simulink model "TST_AdvancedStateflowLoops4"  (Simulink 7.8)
settings: Solver=FixedStepDiscrete  StartTime=0.0  StopTime=10.0  FixedStep=0.02  RelTol=1e-3
settings Model: Creator=kharthforeign  LastModifiedBy=kharthforeign  BufferReuse=off
settings DataIOCC: SaveOutput=off  SignalLogging=off  SaveTime=off
settings OptimizationCC: BlockReduction=off  ConditionallyExecuteInputs=off  OptimizeBlockIOStorage=off  BufferReuse=off  ExpressionFolding=off  LocalBlockOutputs=off  InitFltsAndDblsToZero=on
settings DebuggingCC: FcnCallInpInsideContextMsg=Use local settings  StrictBusMsg=Warning

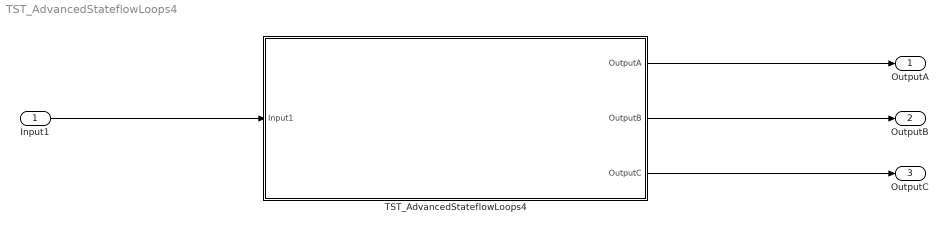
== system TST_AdvancedStateflowLoops4 ==
  Input1 : Inport  OutDataTypeStr=uint32  BusOutputAsStruct=on
  TST_AdvancedStateflowLoops4 : Subsystem  TreatAsAtomicUnit=on
  OutputA : Outport  OutDataTypeStr=double  PortDimensions=1
  OutputB : Outport  Port=2  OutDataTypeStr=double  PortDimensions=1
  OutputC : Outport  Port=3  OutDataTypeStr=double  PortDimensions=1
  wires:
  Input1/1 -> TST_AdvancedStateflowLoops4/1(Input1)
  TST_AdvancedStateflowLoops4/1(OutputA) -> OutputA/1
  TST_AdvancedStateflowLoops4/2(OutputB) -> OutputB/1
  TST_AdvancedStateflowLoops4/3(OutputC) -> OutputC/1

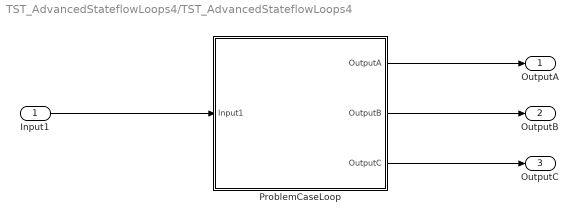
== system TST_AdvancedStateflowLoops4/TST_AdvancedStateflowLoops4 ==
  Input1 : Inport  OutDataTypeStr=uint32  BusOutputAsStruct=on
  ProblemCaseLoop : Stateflow chart  TreatAsAtomicUnit=on
  OutputA : Outport  OutDataTypeStr=double  PortDimensions=1
  OutputB : Outport  Port=2  OutDataTypeStr=double  PortDimensions=1
  OutputC : Outport  Port=3  OutDataTypeStr=double  PortDimensions=1
  wires:
  ProblemCaseLoop/1(OutputA) -> OutputA/1
  ProblemCaseLoop/2(OutputB) -> OutputB/1
  ProblemCaseLoop/3(OutputC) -> OutputC/1
  Input1/1 -> ProblemCaseLoop/1(Input1)

== stateflow chart TST_AdvancedStateflowLoops4/ProblemCaseLoop ==
  note: This flowgraph shows a current problem case for the code-generator,
      | where the first vertex of the loop is not the one with the loop condition
  note: #2
  note: #1
  note: #3
  note: #5
  note: #4
  (junction 9) -> (junction 11) [order 1] : [A]
  (junction 10) -> (junction 9) : {OutputA = 1.0}
  (default) -> (junction 10)
  (junction 11) -> (junction 10) : {OutputA += 2.0}
  (junction 9) -> (junction 12) [order 3]
  (junction 9) -> (junction 13) [order 2] : [B]
  data: Input1 input uint32; OutputA output double =1; OutputB output double =2; OutputC output double =3; Local local uint32 =0; A local boolean; B local boolean; C local boolean; D local boolean
